simulink model "Motor_control_system"  (Simulink 6.0)
settings: Solver=ode45  StartTime=0.0  StopTime=100  RelTol=1e-3
settings Model: LastModifiedBy=student

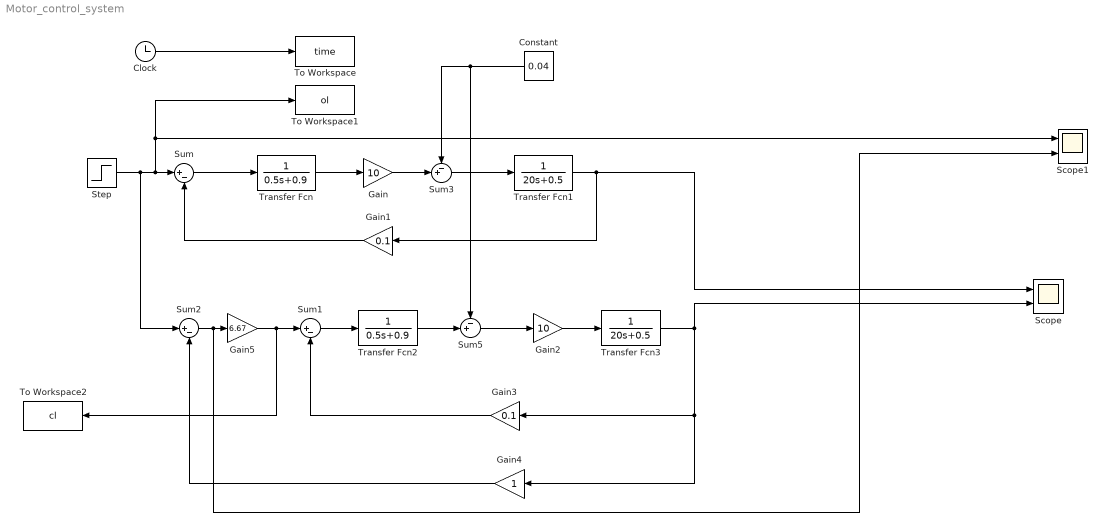
== system Motor_control_system ==
  Clock : Clock
      settings: Decimation=10
  Constant : Constant  Orientation=left  Value=0.04
  Gain : Gain  Gain=10
  Gain1 : Gain  Orientation=left  Gain=0.1
  Gain2 : Gain  Gain=10
  Gain3 : Gain  Orientation=left  Gain=0.1
  Gain4 : Gain  Orientation=left
  Gain5 : Gain  Gain=6.67
  Scope : Scope  NumInputPorts=2
      settings: TimeRange=4  YMin=0~1.3177  YMax=7~2.0377
  Scope1 : Scope  NumInputPorts=2
      settings: TimeRange=4  YMin=0~1.3177  YMax=7~2.0377
  Step : Step  SampleTime=0
  Sum : Sum  Inputs=|+-
  Sum1 : Sum  Inputs=|+-
  Sum2 : Sum  Inputs=|+-
  Sum3 : Sum  Inputs=-+|
  Sum5 : Sum  Inputs=-+|
  To Workspace : ToWorkspace  VariableName=time  SampleTime=-1  SaveFormat=Array
  To Workspace1 : ToWorkspace  VariableName=ol  SampleTime=-1  SaveFormat=Array
  To Workspace2 : ToWorkspace  VariableName=cl  SampleTime=-1  SaveFormat=Array
  Transfer Fcn : TransferFcn  Denominator=[0.5 0.9]
  Transfer Fcn1 : TransferFcn  Denominator=[20 0.5]
  Transfer Fcn2 : TransferFcn  Denominator=[0.5 0.9]
  Transfer Fcn3 : TransferFcn  Denominator=[20 0.5]
  wires:
  Transfer Fcn/1 -> Gain/1
  Sum/1 -> Transfer Fcn/1
  Gain1/1 -> Sum/2
  Step/1 -> Sum2/1, Sum/1, To Workspace1/1, Scope1/1
  Clock/1 -> To Workspace/1
  Gain2/1 -> Transfer Fcn3/1
  Transfer Fcn3/1 -> Gain3/1, Gain4/1, Scope/2
  Sum1/1 -> Transfer Fcn2/1
  Gain3/1 -> Sum1/2
  Gain5/1 -> Sum1/1, To Workspace2/1
  Sum2/1 -> Gain5/1, Scope1/2
  Gain4/1 -> Sum2/2
  Transfer Fcn1/1 -> Gain1/1, Scope/1
  Sum3/1 -> Transfer Fcn1/1
  Gain/1 -> Sum3/2
  Constant/1 -> Sum3/1, Sum5/1
  Transfer Fcn2/1 -> Sum5/2
  Sum5/1 -> Gain2/1
